simulink model "stiffMechanicalSystem"  (R2022b)
settings: Solver=VariableStepAuto  StartTime=0.0  StopTime=10  RelTol=1e-3
settings Model: Creator=bneiswan  LastModifiedBy=bensweet
settings SolverCC: AlgebraicLoopSolver=TrustRegion
settings DebuggingCC: UnconnectedInputMsg=warning  UnconnectedOutputMsg=warning  UnconnectedLineMsg=warning  SFMachineParentedDataDiag=warning
settings ModelReferenceCC: EnableRefExpFcnMdlSchedulingChecks=on
settings RTWCC: DLArmComputeVersion=19.05

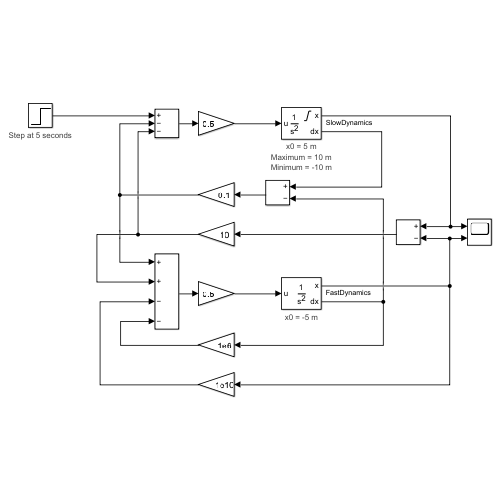
[thumbnail: Simulink's stored preview of the top-level diagram]
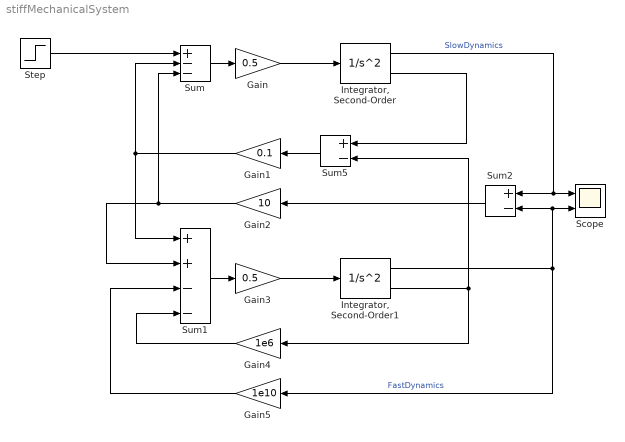
== system stiffMechanicalSystem ==
  Gain : Gain  Gain=0.5
  Gain1 : Gain  Gain=0.1
  Gain2 : Gain  Gain=10
  Gain3 : Gain  Gain=0.5
  Gain4 : Gain  Gain=1e6
  Gain5 : Gain  Gain=1e10
  "Integrator, Second-Order" : SecondOrderIntegrator  ICX=5  LimitX=on  UpperLimitX=10  LowerLimitX=-10
      settings: AttributesFormatString=|
      | x0 = %<ICX> m
      | Maximum = %<UpperLimitX> m
      | Minimum = %<LowerLimitX> m
  "Integrator, Second-Order1" : SecondOrderIntegrator  ICX=-5
      settings: AttributesFormatString=x0 = %<ICX> m
  Scope : Scope  NumInputPorts=2
  Step : Step  Time=5  After=50  SampleTime=0
      settings: AttributesFormatString=Step at %<Time> seconds
  Sum : Sum  Inputs=+--  InputSameDT=on  SaturateOnIntegerOverflow=on  OutDataTypeStr=Inherit: Same as first input
  Sum1 : Sum  Inputs=++--  InputSameDT=on  SaturateOnIntegerOverflow=on  OutDataTypeStr=Inherit: Same as first input
  Sum2 : Sum  Inputs=+-  InputSameDT=on  SaturateOnIntegerOverflow=on  OutDataTypeStr=Inherit: Same as first input
  Sum5 : Sum  Inputs=+-  InputSameDT=on  SaturateOnIntegerOverflow=on  OutDataTypeStr=Inherit: Same as first input
  wires:
  Sum1/1 -> Gain3/1
  Gain1/1 -> Sum1/1, Sum/2
  Gain4/1 -> Sum1/4
  Sum/1 -> Gain/1
  Gain5/1 -> Sum1/3
  Sum2/1 -> Gain2/1
  Gain3/1 -> "Integrator, Second-Order1"/1
  "Integrator, Second-Order1"/1 -> Gain5/1, Sum2/2, Scope/2  "FastDynamics"
  "Integrator, Second-Order"/1 -> Sum2/1, Scope/1  "SlowDynamics"
  Gain2/1 -> Sum1/2, Sum/3
  Gain/1 -> "Integrator, Second-Order"/1
  Sum5/1 -> Gain1/1
  "Integrator, Second-Order"/2 -> Sum5/1
  "Integrator, Second-Order1"/2 -> Sum5/2, Gain4/1
  Step/1 -> Sum/1
